simulink model "MultiVisualLocalizationAgent"  (R2024b)
settings: Solver=FixedStepAuto  StartTime=0.0  StopTime=inf  FixedStep=0.005  RelTol=1e-3  EnableMultiTasking=on
undefined symbols (not defined in the file or in its folder): gray, Sim3dSensor
libraries: eeGeneralControl x7, robotcorelib x7, dspstat3 x3, sim3dcameralib x2, uavsim3dlib x2, sim3dlib x1, uavutilslib x1
settings Model: Creator=The MathWorks, Inc.  LastModifiedBy=vince
settings SolverCC: AlgebraicLoopSolver=TrustRegion  PositivePriorityOrder=on  AutoInsertRateTranBlk=on  MaxZcPerStep=1
settings OptimizationCC: DefaultParameterBehavior=Inlined  EnhancedBackFolding=on  PassReuseOutputArgsAs=Individual arguments  ZeroExternalMemoryAtStartup=off  ZeroInternalMemoryAtStartup=off  MaxStackSize=200000  OptimizeBlockOrder=speed  DifferentSizesBufferReuse=on  OptimizationCustomize=off  EfficientTunableParamExpr=on
settings DebuggingCC: ParameterTunabilityLossMsg=error  UnconnectedInputMsg=warning  UnconnectedOutputMsg=warning  UnconnectedLineMsg=warning  SymbolicDimsDataTypeCodeGenerationDiagnostic=none
settings HardwareCC: ProdBitPerPointer=32  ProdBitPerSizeT=32  ProdBitPerPtrDiffT=32  ProdLargestAtomicInteger=Long  ProdLargestAtomicFloat=Double  ProdWordSize=32  ProdLongLongMode=on  ProdHWDeviceType=ARM Compatible->ARM Cortex-A (32-bit)
settings ModelReferenceCC: EnableRefExpFcnMdlSchedulingChecks=on
settings RTWCC: Description=Embedded Coder  SystemTargetFile=ert.tlc  HardwareBoard=Raspberry Pi  TLCOptions="-aInlineSetEventsForThisBaseRateFcn=TLC_FALSE -aSuppressMultiTaskScheduler=TLC_FALSE  -aRateBasedStepFcn=0"  TemplateMakefile=ert_default_tmf  Toolchain=GNU GCC Embedded Linux  BuildConfiguration=Faster Runs  GPUComputeCapability=3.5  DLArmComputeVersion=19.05
settings CodeAppCC: ForceParamTrailComments=on  IgnoreCustomStorageClasses=off  OperatorAnnotations=on  SimulinkDataObjDesc=on  SFDataObjDesc=on  InsertBlockDesc=on
settings ERTTargetCC: CodeReplacementLibrary=ARM Cortex-A CMSIS  SupportVariableSizeSignals=on  ExtModeTransport=2  ExtModeStaticAlloc=on  ExtModeMexFile=ext_xcp  ExtModeIntrfLevel=Level2 - Open

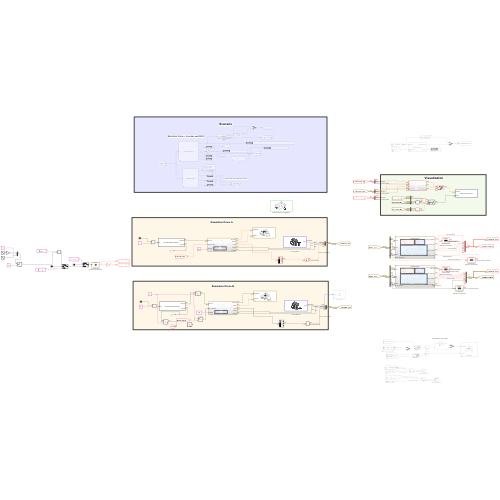
[thumbnail: Simulink's stored preview of the top-level diagram]
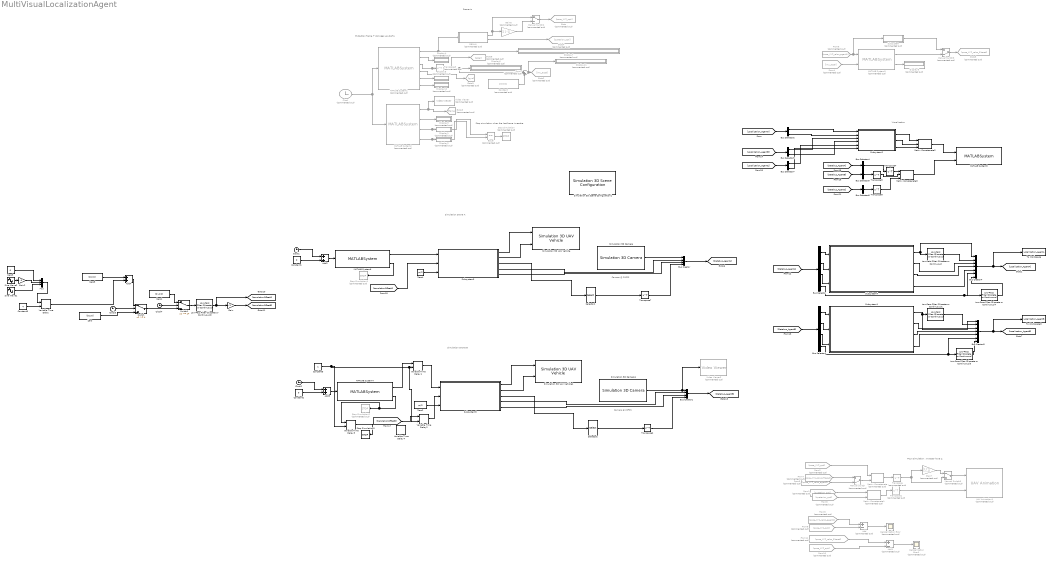
== system MultiVisualLocalizationAgent ==
  note: Stop simulation when the last frame is reache
  note: Pour Simulation : Inverser l'axe Z
  note: Extraction frame + données uavDATA
  note: Scenario
  note: Visualization
  note: Camera @ 20FPS
  note: Simulation Drone A
  note: Camera @ 20FPS
  note: Simulation Drone B
  Add : Sum  Commented=on  Inputs=+-
  Add1 : Sum  Commented=on  Inputs=+-
  Add2 : Sum
  Add3 : Sum
  Add4 : Sum
  Bus Creator : BusCreator  Inputs=4
  Bus Creator1 : BusCreator  Inputs=4
  Bus Creator3 : BusCreator  Inputs=7
  Bus Creator4 : BusCreator  Inputs=7
  Bus Selector : BusSelector  OutputSignals=accel,gyro,frame,Pose_XYZ_GroundTruth
  Bus Selector1 : BusSelector  OutputSignals=accel,gyro,frame,Pose_XYZ_GroundTruth
  Bus Selector2 : BusSelector  OutputSignals=Rotation_Mat_Reloc,Pose_XYZ_Kalman_Filtered
  Bus Selector3 : BusSelector  OutputSignals=Rotation_Mat_Reloc,Pose_XYZ_Kalman_Filtered
  Bus Selector4 : BusSelector  OutputSignals=Pose_XYZ_GroundTruth
  Bus Selector5 : BusSelector  OutputSignals=Pose_XYZ_GroundTruth
  Bus Selector7 : BusSelector  OutputSignals=Rotation_Mat_Reloc,Pose_XYZ_Kalman_Filtered
  Bus Selector8 : BusSelector  OutputSignals=Pose_XYZ_GroundTruth
  Clock : Clock  Commented=on
  Clock{1..4} (4 alike) : Clock
  Constant : Constant  Commented=on  Value=[0 0 0]
  Constant1 : Constant  Value=0
  Constant2 : Constant  Value=0
  Constant3 : Constant  Value=4
  Constant5 : Constant
  DEMUX : Subsystem  Commented=on
  Display{1..8,10..11} (10 alike) : Display  Commented=on
  Equal : RelationalOperator  Commented=on  Operator===  OutDataTypeStr=boolean  RndMeth=Simplest  InputSameDT=off
  From1 : From  Commented=on  GotoTag=quaterion_opti
  From10 : From  Commented=on  GotoTag=pose_XYZ_opti
  From11 : From  Commented=on  GotoTag=pose_XYZ_reloc_filtered
  From2 : From  Commented=on  GotoTag=pose_XYZ_opti
  From3 : From  Commented=on  GotoTag=pose_XYZ_reloc_agent1
  From4 : From  Commented=on  GotoTag=imu_accel
  From5 : From  Commented=on  GotoTag=quaterion_opti
  From6 : From  Commented=on  GotoTag=pose_XYZ_reloc_agent1
  From7 : From  Commented=on  GotoTag=pose_XYZ_reloc_filtered
  From8 : From  Commented=on  GotoTag=pose_XYZ_opti
  From9 : From  Commented=on  GotoTag=pose_XYZ_reloc_agent1
  Gain : Gain  Gain=-1
  Gain2 : Gain  Gain=-1
  Gain6 : Gain  Commented=on  Gain=[1 1 -1]
  Gain7 : Gain  Commented=on  Gain=[1 1 -1; 1 1 -1]
  Goto : Goto  Commented=on  GotoTag=pose_XYZ_opti
  Goto2 : Goto  Commented=on  GotoTag=imu_accel
  Goto3 : Goto  Commented=on  GotoTag=frame
  Goto4 : Goto  Commented=on  GotoTag=quaterion_opti
  Goto5 : Goto  Commented=on  GotoTag=pose_XYZ_reloc_filtered
  Goto8 : Goto  Commented=on  GotoTag=accel
  Goto9 : Goto  Commented=on  GotoTag=gyro
  Low-Pass Filter (Discrete or Continuous){,1,3..4} (4 alike) : eeGeneralControl/Low-Pass Filter (Discrete or Continuous)  K=1  T=0.5  B=inf  A=-inf  init_option=Inherited from block input  x0=0  Ts=-1
  Low-Pass Filter (Discrete or Continuous)2 : eeGeneralControl/Low-Pass Filter (Discrete or Continuous)  K=1  T=1  B=inf  A=-inf  init_option=Inherited from block input  x0=0  Ts=-1
  MATLAB System1 : MATLABSystem  Commented=on  System=GTruthPlayerSystem  groundTruthFile=C:\Users\vince\Documents\SEN5\CollaborativeSLAM\Scenarios\7\uavData.mat  SimulateUsing=Interpreted execution
      mask Type: GTruthPlayerSystem
      mask Display: disp('GTruthPlayerSystem');
  MATLAB System2 : MATLABSystem  Commented=on  System=ImagePlayerSystem  imageFolder=C:\Users\vince\Documents\SEN5\CollaborativeSLAM\Scenarios\7\images  cameraSize=[720,1280, 1]  groundTruthFile=C:\Users\vince\Documents\SEN5\CollaborativeSLAM\Scenarios\7\uavData.mat  SimulateUsing=Interpreted execution
      mask Type: ImagePlayerSystem
      mask Display: disp('ImagePlayerSystem');
  MATLAB System3 : MATLABSystem  Commented=on  System=PositionAccelFilter  maxPositionJump=0.2  maxAcceleration=10.0  windowSize=5  alpha=0.1  SimulateUsing=Code generation
      mask Type: PositionAccelFilter
      mask Display:
      | disp('PositionAccelFilter');
      | port_label('input',1,'position');
      | port_label('input',2,'acceleration');
      | port_label('output',1,'filteredPosition');
      | port_label('output',2,'isJump');
  MATLAB System4 : MATLABSystem  System=SmoothBasicWaypointManager  ScenariosDirectory=C:\Users\vince\Documents\SEN5\CollaborativeSLAM\Scenarios  ScenarioName=6  StepTime=0.01  SimulateUsing=Interpreted execution
      mask Type: SmoothBasicWaypointManager
      mask Display:
      | disp('SmoothBasicWaypointManager');
      | port_label('input',1,'time');
      | port_label('output',1,'waypoint');
      | port_label('output',2,'finished');
  MATLAB System5 : MATLABSystem  System=HelperVisualizationSystem  XLim=[-10 60]  YLim=[-10 10]  ZLim=[-10 10]  SampleTime=-1  ScenariosDirectory=C:\Users\vince\Documents\SEN5\CollaborativeSLAM\Scenarios  ScenarioName=8  NumberOfPoses=3  SimulateUsing=Interpreted execution
      mask Type: HelperVisualizationSystem
      mask Display:
      | disp('HelperVisualizationSystem');
      | port_label('input',1,'TformID');
      | port_label('input',2,'Gtruth');
  MATLAB System6 : MATLABSystem  System=SmoothBasicWaypointManager  ScenariosDirectory=C:\Users\vince\Documents\SEN5\CollaborativeSLAM\Scenarios  ScenarioName=6  StepTime=0.01  SimulateUsing=Interpreted execution
      mask Type: SmoothBasicWaypointManager
      mask Display:
      | disp('SmoothBasicWaypointManager');
      | port_label('input',1,'time');
      | port_label('output',1,'waypoint');
      | port_label('output',2,'finished');
  Manual Switch : ManualSwitch  Commented=on  CurrentSetting=0
  Manual Switch2 : ManualSwitch  Commented=on
  Manual Switch3 : ManualSwitch  Commented=on  CurrentSetting=0
  Manual Switch5 : ManualSwitch  Commented=on
  Matrix Concatenate : Concatenate  Commented=on  Mode=Multidimensional array  ConcatenateDimension=2
  Matrix Concatenate1 : Concatenate  Commented=on  Mode=Multidimensional array  ConcatenateDimension=2
  Matrix Concatenate2 : Concatenate  NumInputs=3  Mode=Multidimensional array  ConcatenateDimension=2
  Matrix Concatenate3 : Concatenate  NumInputs=3  Mode=Multidimensional array  ConcatenateDimension=2
  Mux : Mux  Inputs=3
  Relocalization Error : Scope  Commented=on
  Relocalization Error1 : Scope  Commented=on
  Selector1 : Selector  InputPortWidth=7  IndexOptions=Index vector (dialog)  Indices=[1 2 3]  OutputSizes=1
  Selector2 : Selector  InputPortWidth=7  IndexOptions=Index vector (dialog)  Indices=[1 2 3]  OutputSizes=1
  Simulation 3D Camera : sim3dcameralib/Simulation 3D Camera  Priority=1  sensorTag=Sim3dSensor�  sensorId=1  sensorName=Sim3dSensor�  vehTagList={'Scene Origin';'SimulinkVehicle1'}  vehTag=SimulinkVehicle1  mountLoc=Origin  offsetFlag=on  tmountOffset=[0.1, 0, 0.1]  extTmount=off  rmountOffset=[0, 0, 0]  extRmount=off  FocalLength=[1109, 1109]  OpticalCenter=[640, 360]  ImageSize=[720, 1280]  RadialDistortion=[0, 0]  TangentialDistortion=[0, 0]  SensorSkew=0  DepthOutportEnabled=off  SemanticOutportEnabled=off  TransformOutportEnabled=off  SampleTime=1/20  mountPoint=[0.1 0 0.1]  mountOrientation=[0 0 0]  aMode=3  ID=1
      settings: LibrarySourceBlock=drivingsim3d/Simulation 3D Camera
  Simulation 3D Camera1 : sim3dcameralib/Simulation 3D Camera  Priority=1  sensorTag=Sim3dSensor�  sensorId=2  sensorName=Sim3dSensor�  vehTagList={'Scene Origin';'SimulinkVehicle1';'SimulinkVehicle2'}  vehTag=SimulinkVehicle2  mountLoc=Origin  offsetFlag=on  tmountOffset=[0.1, 0, 0.1]  extTmount=off  rmountOffset=[0, 0, 0]  extRmount=off  FocalLength=[1109, 1109]  OpticalCenter=[640, 360]  ImageSize=[720, 1280]  RadialDistortion=[0, 0]  TangentialDistortion=[0, 0]  SensorSkew=0  DepthOutportEnabled=off  SemanticOutportEnabled=off  TransformOutportEnabled=off  SampleTime=1/20  mountPoint=[0.1 0 0.1]  mountOrientation=[0 0 0]  aMode=3  ID=2
      settings: LibrarySourceBlock=drivingsim3d/Simulation 3D Camera
  Simulation 3D Scene Configuration1 : sim3dlib/Simulation 3D Scene Configuration  Priority=0  ProjectFormat=Default Scenes  SceneDesc=US city block  ProjectName=C:\Program Files\MATLAB\R2024b\toolbox\shared\sim3d_projects\automotive_project_windows\UE\WindowsNoEditor\VehicleSimulation.exe  ScenePath=/Game/Maps/USCityBlock  EnableOpenDRIVE=off  vehTagList={'Custom';'Scene Origin';'SimulinkVehicle1';'SimulinkVehicle2';'SimulinkVehicle3'}  vehTag=SimulinkVehicle1  FreeCameraInitialTranslation=[0, 0, 0]  FreeCameraDefaultInitialTranslation=[-6, 0, 2]  FreeCameraInitialRotation=[0, 0, 0]  FreeCameraDefaultInitialRotation=[0, -15, 0]  OpVisEn=off  Ts=1/100  EnableWindow=off  EnableRemoteAccess=off  EnableWeather=off  SunAzimuth=90  SunAltitude=40.0  EnableGeospatialSun=off  Latitude=0  Longitude=0  Date=2023-01-01  Time=10:30:00  GeoTimeZone=-5.0  SunDaylightSaving=off  wind=1  clouds=10  EnableVolumetricClouds=off  CloudCoverage=0  CloudAltitude=6  fog=0  rain=0  RaindropsEffect=off  SnowDensity=0  EnableGeospatial=off  UseTrueOrigin=off  OriginHeight=200  OriginLatitude=40.744652  OriginLongitude=-73.988864  MapStyle=Aerial  AdditionalAssetIDs=[]  UseAdvancedSunSky=off  SolarTime=11  TimeZone=-5  Day=21  Month=9  Year=2022  UseDaylightSavingTime=on  DSTStartDay=10  DSTStartMonth=3  DSTEndDay=3  DSTEndMonth=11  DSTSwitchHour=2  sensorTag=MainCamera1  sensorId=1  sensorName=MainCamera1  mountLoc=Origin  offsetFlag=off  tmountOffset=[0, 0, 0]  rmountOffset=[0, 0, 0]  HorizontalResolution=1280  VerticalResolution=720  HorizontalFOV=60  mountPoint=[0 0 0]  mountOrientation=[0 0 0]  aMode=4  ID=1  GeoTrigger=Inactive
      settings: LibrarySourceBlock=uavsim3dlib/Simulation 3D Scene Configuration
  Simulation 3D UAV Vehicle : uavsim3dlib/Simulation 3D UAV Vehicle  Priority=-1  Mesh=Quadrotor  MeshPath=/MathWorksUAVContent/UAVs/HexaRotorUAV/HexaRotor.HexaRotor  Color=Black  ActorName=SimulinkVehicle1  UseGlobalFrame=off  InitialTranslation=[0 0 0]  InitialRotation=[0 0 0]  InitialTranslationGlobal=[0 0 0]  InitialGeoOrigin=[0 0 0]  InitialRotationGlobal=[0 0 0]  SampleTime=1/100  ActorType=SimulinkVehicle  ID=1  aMode=4  ActorTag=SimulinkVehicle1
  Simulation 3D UAV Vehicle1 : uavsim3dlib/Simulation 3D UAV Vehicle  Priority=-1  Mesh=Quadrotor  MeshPath=/MathWorksUAVContent/UAVs/HexaRotorUAV/HexaRotor.HexaRotor  Color=Black  ActorName=SimulinkVehicle2  UseGlobalFrame=off  InitialTranslation=[0 -2 0]  InitialRotation=[0 0 0]  InitialTranslationGlobal=[0 0 0]  InitialGeoOrigin=[0 0 0]  InitialRotationGlobal=[0 0 0]  SampleTime=1/100  ActorType=SimulinkVehicle  ID=2  aMode=4  ActorTag=SimulinkVehicle2
  Sine Wave1 : Sin  Frequency=2*pi/20  SampleTime=0
  Sine Wave2 : Sin  Amplitude=4  Frequency=2*pi/40  SampleTime=0
  Stop Simulation : Stop  Commented=on
  Stop Simulation1 : Stop  Commented=on
  Stop Simulation2 : Stop  Commented=on
  Stop Simulation3 : Stop
  Subsystem : Subsystem  Commented=on
  Subsystem1 : Subsystem  ReferencedSubsystem=LocalizationSystem
  Subsystem2 : Subsystem
  Subsystem3 : Subsystem
  Subsystem4 : Subsystem  ReferencedSubsystem=LocalizationSystem
  Subsystem5 : Subsystem
  Sum1 : Sum  Commented=on  Inputs=|++
  Switch : Switch  Threshold=4  SaturateOnIntegerOverflow=off  InputSameDT=off
  Switch1 : Switch  Threshold=14  SaturateOnIntegerOverflow=off  InputSameDT=off
  To Workspace : ToWorkspace  VariableName=Localization_AgentA  SaveFormat=Timeseries  SampleTime=-1
  To Workspace3 : ToWorkspace  VariableName=Localization_AgentB  SaveFormat=Timeseries  SampleTime=-1
  Transpose : Math  Commented=on  Operator=transpose
  Transpose1 : Math  Commented=on  Operator=transpose
  Transpose{2,4..5,7..8} (5 alike) : Math  Operator=transpose
  Transpose3 : Math  Commented=on  Operator=transpose
  UAV Animation1 : uavutilslib/UAV Animation  Commented=on  NumUAV=2  DynamicUAVConfig=off  UAVType=Multirotor  UAVSize=0.1  UAVColor=[1 0 0]  UAVTrajectoryAlpha=1  InertialZDirection=Down  RotationFormat=Quaternion  DrawMarkers=off  SampleTime=-1
  Variable Time Delay{,1..4} (5 alike) : VariableTransportDelay  MaximumDelay=10
  Video Viewer : VideoViewer  Commented=on  colormapValue=gray(256)  FigPos=[184.333333333333 766.666666666667 706 510]
  Video Viewer2 : VideoViewer  Commented=on  FigPos=[1 1030 1920 930]
  Zero : Constant  Value=[0;2;0]  OutDataTypeStr=Inherit: Inherit via back propagation
  Zero1 : Constant  Value=[0;-2;0]  OutDataTypeStr=Inherit: Inherit via back propagation
  Zero2 : Constant  Value=-pi/2  OutDataTypeStr=Inherit: Inherit via back propagation
  Zero3 : Constant  Value=0  OutDataTypeStr=Inherit: Inherit via back propagation
  Zero4 : Constant  Value=-pi/2  OutDataTypeStr=Inherit: Inherit via back propagation
  Zero5 : Constant  Value=[0;2;0]  OutDataTypeStr=Inherit: Inherit via back propagation
  wires:
  MATLAB System2/1 -> Goto3/1, Video Viewer/1
  MATLAB System2/3 -> Equal/1, Display1/1
  Clock/1 -> MATLAB System2/1, MATLAB System1/1
  MATLAB System2/4 -> Equal/2, Display2/1
  MATLAB System2/2 -> Display3/1
  MATLAB System1/1 -> Display7/1, DEMUX/1(pose_refopti_gtruth)
  Matrix Concatenate/1 -> Transpose/1
  Matrix Concatenate1/1 -> Transpose1/1
  Transpose/1 -> Gain7/1, Manual Switch5/2
  Transpose1/1 -> UAV Animation1/2
  From3/1 -> Manual Switch/2
  DEMUX/1(XYZ_gtruth) -> Manual Switch2/1, Gain6/1
  MATLAB System1/2 -> Display4/1
  MATLAB System1/5 -> Display5/1
  MATLAB System1/6 -> Display10/1
  MATLAB System1/3 -> Goto8/1, Transpose3/1
  DEMUX/2(quaterion_gtruth) -> Goto4/1
  From1/1 -> Matrix Concatenate1/1
  From5/1 -> Matrix Concatenate1/2
  From4/1 -> MATLAB System3/2
  From6/1 -> Subsystem/1(In1), MATLAB System3/1
  From7/1 -> Manual Switch/1
  Manual Switch/1 -> Matrix Concatenate/2
  Transpose3/1 -> Sum1/1, Display6/1
  MATLAB System3/2 -> Display8/1
  Constant/1 -> Sum1/2
  Sum1/1 -> Display11/1, Goto2/1
  MATLAB System3/1 -> Manual Switch3/2
  Subsystem/1(Out1) -> Manual Switch3/1
  From2/1 -> Matrix Concatenate/1
  Gain6/1 -> Manual Switch2/2
  Manual Switch2/1 -> Goto/1
  From8/1 -> Add/2  "Real_Pose_XYZ"
  Add/1 -> Relocalization Error/1  "Relocalization Error"
  From9/1 -> Add/1  "Estimated_Pose_XYZ"
  Add1/1 -> Relocalization Error1/1  "Filtered Relocalization Error"
  From10/1 -> Add1/2  "Real_Pose_XYZ"
  From11/1 -> Add1/1  "Estimated_Pose_XYZ_Filtered"
  Manual Switch3/1 -> Goto5/1
  Equal/1 -> Stop Simulation/1
  Manual Switch5/1 -> UAV Animation1/1
  Gain7/1 -> Manual Switch5/1
  MATLAB System1/4 -> Goto9/1
  Bus Selector2/1 -> Subsystem2/1(In1)  "<Rotation_Mat_Reloc>"
  Bus Selector2/2 -> Subsystem2/2(In2)  "<Pose_XYZ_Kalman_Filtered>"
  Subsystem2/1(Out1) -> Matrix Concatenate2/1
  Subsystem2/2(Out2) -> Matrix Concatenate2/2
  Clock1/1 -> Add2/1
  Add2/1 -> MATLAB System6/1
  Subsystem3/4(accData) -> Bus Creator/2  "accel"
  MATLAB System6/1 -> Subsystem3/1(waypoint)
  [translationOffsetA] -> Subsystem3/2(translationOffset)
  Subsystem3/1(Translation) -> Simulation 3D UAV Vehicle/1
  Subsystem3/3(gTruth) -> Selector1/1
  Zero4/1 -> Subsystem3/3(initialYaw)
  Subsystem3/2(Rotation) -> Simulation 3D UAV Vehicle/2
  MATLAB System6/2 -> Stop Simulation1/1
  Constant1/1 -> Add2/2
  Subsystem3/5(gyroData) -> Bus Creator/3  "gyro"
  Simulation 3D Camera/1 -> Bus Creator/1  "frame"
  Bus Selector3/2 -> Subsystem2/4(In4)  "<Pose_XYZ_Kalman_Filtered>"
  Bus Selector3/1 -> Subsystem2/3(In3)  "<Rotation_Mat_Reloc>"
  Selector1/1 -> Transpose7/1
  Transpose7/1 -> Bus Creator/4  "Pose_XYZ_GroundTruth"
  Matrix Concatenate3/1 -> MATLAB System5/2
  Low-Pass Filter (Discrete or Continuous)/1 -> Bus Creator4/2  "Pose_XYZ_Kalman_Filtered"
  Subsystem4/1 -> Low-Pass Filter (Discrete or Continuous)/1, Bus Creator4/1  "Pose_XYZ_Kalman"
  Subsystem4/3 -> Bus Creator4/4  "Pose_XYZ_Reloc"
  Subsystem4/4 -> Bus Creator4/5  "Rotation_Mat_Reloc"
  Bus Selector/3 -> Subsystem4/3  "<frame>"
  Bus Selector/2 -> Subsystem4/2  "<gyro>"
  Bus Selector/1 -> Subsystem4/1  "<accel>"
  Bus Creator/1 -> [Databus_AgentA]
  [Databus_AgentA] -> Bus Selector/1
  Bus Selector1/2 -> Subsystem1/2  "<gyro>"
  Bus Selector1/3 -> Subsystem1/3  "<frame>"
  [Databus_AgentB] -> Bus Selector1/1
  Bus Selector1/1 -> Subsystem1/1  "<accel>"
  Bus Creator1/1 -> [Databus_AgentB]
  Subsystem5/4(accData) -> Bus Creator1/2  "accel"
  Subsystem5/3(gTruth) -> Selector2/1
  Clock2/1 -> Add3/1
  Subsystem5/5(gyroData) -> Bus Creator1/3  "gyro"
  Subsystem5/2(Rotation) -> Simulation 3D UAV Vehicle1/2
  MATLAB System4/2 -> Variable Time Delay3/1, Stop Simulation2/1
  Add3/1 -> MATLAB System4/1
  Zero2/1 -> Subsystem5/3(initialYaw)
  Constant2/1 -> Add3/2
  MATLAB System4/1 -> Variable Time Delay1/1
  Transpose2/1 -> Bus Creator1/4  "Pose_XYZ_GroundTruth"
  Subsystem5/1(Translation) -> Simulation 3D UAV Vehicle1/1
  Selector2/1 -> Transpose2/1
  Bus Creator4/1 -> To Workspace/1, [Localization_AgentA]  "AgentA"
  Bus Creator3/1 -> To Workspace3/1, [Localization_AgentB]  "AgentB"
  Subsystem1/4 -> Bus Creator3/5  "Rotation_Mat_Reloc"
  Subsystem1/3 -> Bus Creator3/4  "Pose_XYZ_Reloc"
  Low-Pass Filter (Discrete or Continuous)1/1 -> Bus Creator3/2  "Pose_XYZ_Kalman_Filtered"
  Subsystem1/1 -> Bus Creator3/1, Low-Pass Filter (Discrete or Continuous)1/1  "Pose_XYZ_Kalman"
  [Localization_AgentA] -> Bus Selector2/1
  [Localization_AgentB] -> Bus Selector3/1
  [Databus_AgentA] -> Bus Selector4/1
  Bus Selector4/1 -> Transpose4/1  "<Pose_XYZ_GroundTruth>"
  [Databus_AgentB] -> Bus Selector5/1
  Bus Selector5/1 -> Transpose5/1  "<Pose_XYZ_GroundTruth>"
  Transpose4/1 -> Matrix Concatenate3/1
  Transpose5/1 -> Matrix Concatenate3/2
  Matrix Concatenate2/1 -> MATLAB System5/1
  Subsystem1/2 -> Bus Creator3/3
  Subsystem4/2 -> Bus Creator4/3
  Clock3/1 -> Switch/2
  Zero/1 -> Switch/3
  Switch1/1 -> Low-Pass Filter (Discrete or Continuous)2/1
  Switch/1 -> Switch1/3
  Clock4/1 -> Switch1/2
  Zero1/1 -> Switch1/1
  Sine Wave1/1 -> Mux/3
  Zero3/1 -> Mux/1
  Zero5/1 -> Add4/1
  Add4/1 -> Switch/1
  Low-Pass Filter (Discrete or Continuous)2/1 -> [translationOffsetA], Gain/1
  Mux/1 -> Variable Time Delay/1
  Gain2/1 -> Mux/2
  Gain/1 -> [translationOffsetB]
  Sine Wave2/1 -> Gain2/1
  Constant3/1 -> Variable Time Delay/2
  Variable Time Delay/1 -> Add4/2
  Bus Selector1/4 -> Bus Creator3/6, Low-Pass Filter (Discrete or Continuous)3/1  "<Pose_XYZ_GroundTruth>"
  Low-Pass Filter (Discrete or Continuous)3/1 -> Bus Creator3/7  "Pose_XYZ_GroundTruth_Filtered"
  Bus Selector/4 -> Low-Pass Filter (Discrete or Continuous)4/1, Bus Creator4/6  "<Pose_XYZ_GroundTruth>"
  Low-Pass Filter (Discrete or Continuous)4/1 -> Bus Creator4/7  "Pose_XYZ_GroundTruth_Filtered"
  [translationOffsetB] -> Variable Time Delay2/1
  Variable Time Delay2/1 -> Subsystem5/2(translationOffset)
  Variable Time Delay1/1 -> Subsystem5/1(waypoint)
  Constant5/1 -> Variable Time Delay2/2, Variable Time Delay1/2, Variable Time Delay3/2
  Simulation 3D Camera1/1 -> Video Viewer2/1, Bus Creator1/1  "frame"
  Variable Time Delay3/1 -> Stop Simulation3/1
  [Localization_AgentC] -> Bus Selector7/1
  Bus Selector7/1 -> Subsystem2/5(In5)  "<Rotation_Mat_Reloc>"
  Bus Selector7/2 -> Subsystem2/6(In6)  "<Pose_XYZ_Kalman_Filtered>"
  Subsystem2/3(Out3) -> Matrix Concatenate2/3
  [Databus_AgentC] -> Bus Selector8/1
  Transpose8/1 -> Matrix Concatenate3/3
  Bus Selector8/1 -> Transpose8/1  "<Pose_XYZ_GroundTruth>"

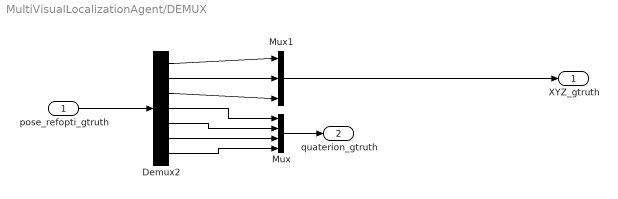
== system MultiVisualLocalizationAgent/DEMUX ==
  pose_refopti_gtruth : Inport
  Demux2 : Demux  Outputs=7
  Mux : Mux
  Mux1 : Mux  Inputs=3
  XYZ_gtruth : Outport
  quaterion_gtruth : Outport  Port=2
  wires:
  Mux/1 -> quaterion_gtruth/1
  Demux2/2 -> Mux1/2
  Demux2/5 -> Mux/2
  Mux1/1 -> XYZ_gtruth/1
  Demux2/3 -> Mux1/3
  Demux2/4 -> Mux/1
  pose_refopti_gtruth/1 -> Demux2/1
  Demux2/7 -> Mux/4
  Demux2/6 -> Mux/3
  Demux2/1 -> Mux1/1

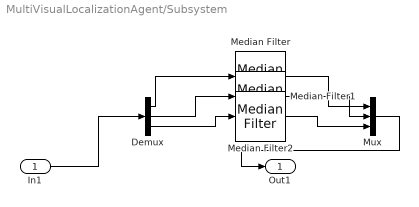
== system MultiVisualLocalizationAgent/Subsystem ==
  In1 : Inport
  Demux : Demux  Outputs=3
  Median Filter : dspstat3/Median Filter  WindowLength=2  SimulateUsing=Interpreted execution
  Median Filter1 : dspstat3/Median Filter  WindowLength=2  SimulateUsing=Interpreted execution
  Median Filter2 : dspstat3/Median Filter  WindowLength=2  SimulateUsing=Interpreted execution
  Mux : Mux  Inputs=3
  Out1 : Outport  PortDimensions=[3 1]
  wires:
  Median Filter2/1 -> Mux/3
  In1/1 -> Demux/1
  Demux/3 -> Median Filter2/1
  Mux/1 -> Out1/1
  Demux/2 -> Median Filter1/1
  Demux/1 -> Median Filter/1
  Median Filter1/1 -> Mux/2
  Median Filter/1 -> Mux/1

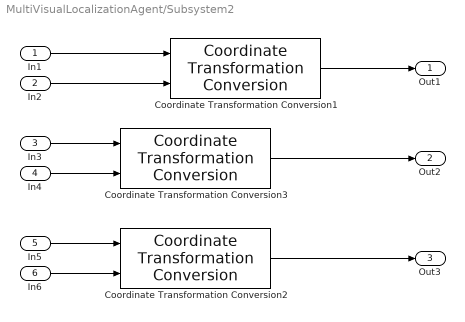
== system MultiVisualLocalizationAgent/Subsystem2 ==
  In1 : Inport
  In2 : Inport  Port=2
  In3 : Inport  Port=3
  In4 : Inport  Port=4
  In5 : Inport  Port=5
  In6 : Inport  Port=6
  Coordinate Transformation Conversion1 : robotcorelib/Coordinate Transformation Conversion  InputRepresentation=Rotation Matrix  InputEulerSequence=ZYX  ShowTrVecInputPort=on  OutputRepresentation=Homogeneous Transformation  OutputEulerSequence=ZYX  ShowTrVecOutputPort=on  SimulateUsing=Code generation
      settings: LibrarySourceBlock=navlib/Utilities/Coordinate Transformation Conversion
  Coordinate Transformation Conversion2 : robotcorelib/Coordinate Transformation Conversion  InputRepresentation=Rotation Matrix  InputEulerSequence=ZYX  ShowTrVecInputPort=on  OutputRepresentation=Homogeneous Transformation  OutputEulerSequence=ZYX  ShowTrVecOutputPort=on  SimulateUsing=Code generation
      settings: LibrarySourceBlock=navlib/Utilities/Coordinate Transformation Conversion
  Coordinate Transformation Conversion3 : robotcorelib/Coordinate Transformation Conversion  InputRepresentation=Rotation Matrix  InputEulerSequence=ZYX  ShowTrVecInputPort=on  OutputRepresentation=Homogeneous Transformation  OutputEulerSequence=ZYX  ShowTrVecOutputPort=on  SimulateUsing=Code generation
      settings: LibrarySourceBlock=navlib/Utilities/Coordinate Transformation Conversion
  Out1 : Outport
  Out2 : Outport  Port=2
  Out3 : Outport  Port=3
  wires:
  Coordinate Transformation Conversion3/1 -> Out2/1
  In3/1 -> Coordinate Transformation Conversion3/1
  Coordinate Transformation Conversion1/1 -> Out1/1
  In1/1 -> Coordinate Transformation Conversion1/1
  In4/1 -> Coordinate Transformation Conversion3/2
  In2/1 -> Coordinate Transformation Conversion1/2
  In6/1 -> Coordinate Transformation Conversion2/2
  In5/1 -> Coordinate Transformation Conversion2/1
  Coordinate Transformation Conversion2/1 -> Out3/1

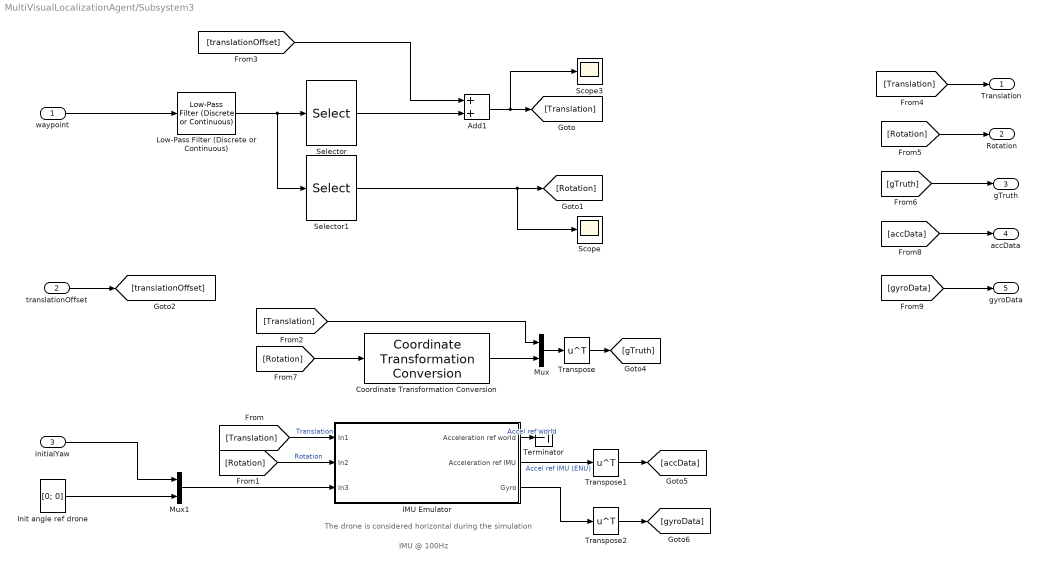
== system MultiVisualLocalizationAgent/Subsystem3 ==
  note: IMU @ 100Hz
  note: The drone is considered horizontal during the simulation
  waypoint : Inport
  translationOffset : Inport  Port=2
  initialYaw : Inport  Port=3
  Add1 : Sum
  Coordinate Transformation Conversion : robotcorelib/Coordinate Transformation Conversion  InputRepresentation=Euler Angles  InputEulerSequence=ZYX  ShowTrVecInputPort=on  OutputRepresentation=Quaternion  OutputEulerSequence=ZYX  ShowTrVecOutputPort=on  SimulateUsing=Code generation
  IMU Emulator : Subsystem
  Init angle ref drone : Constant  Value=[0; 0]  VectorParams1D=off
  Low-Pass Filter (Discrete or Continuous) : eeGeneralControl/Low-Pass Filter (Discrete or Continuous)  K=1  T=0.5  B=inf  A=-inf  init_option=Inherited from block input  x0=0  Ts=-1
  Mux : Mux  Inputs=2
  Mux1 : Mux  Inputs=2
  Scope : Scope
  Scope3 : Scope
  Selector : Selector  InputPortWidth=6  IndexOptions=Index vector (dialog)  Indices=[1 2 3]  OutputSizes=1
  Selector1 : Selector  InputPortWidth=6  IndexOptions=Index vector (dialog)  Indices=[4 5 6]  OutputSizes=1
  Terminator : Terminator
  Transpose : Math  Operator=transpose
  Transpose1 : Math  Operator=transpose
  Transpose2 : Math  Operator=transpose
  Translation : Outport
  Rotation : Outport  Port=2
  gTruth : Outport  Port=3
  accData : Outport  Port=4
  gyroData : Outport  Port=5
  wires:
  waypoint/1 -> Low-Pass Filter (Discrete or Continuous)/1
  Add1/1 -> Scope3/1, [Translation]
  Transpose2/1 -> [gyroData]
  Selector/1 -> Add1/2
  Init angle ref drone/1 -> Mux1/2
  Selector1/1 -> [Rotation], Scope/1
  IMU Emulator/3(Gyro) -> Transpose2/1
  Coordinate Transformation Conversion/1 -> Mux/2
  IMU Emulator/1(Acceleration ref world) -> Terminator/1  "Accel ref world"
  [translationOffset] -> Add1/1
  Mux/1 -> Transpose/1
  [Rotation] -> Coordinate Transformation Conversion/1
  Transpose1/1 -> [accData]
  Transpose/1 -> [gTruth]
  [Translation] -> Mux/1
  Low-Pass Filter (Discrete or Continuous)/1 -> Selector1/1, Selector/1
  [Rotation] -> IMU Emulator/2(In2)  "Rotation"
  [Translation] -> IMU Emulator/1(In1)  "Translation"
  IMU Emulator/2(Acceleration ref IMU) -> Transpose1/1  "Accel ref IMU (ENU)"
  [Translation] -> Translation/1
  [Rotation] -> Rotation/1
  [gTruth] -> gTruth/1
  [accData] -> accData/1
  [gyroData] -> gyroData/1
  initialYaw/1 -> Mux1/1
  Mux1/1 -> IMU Emulator/3(In3)
  translationOffset/1 -> [translationOffset]

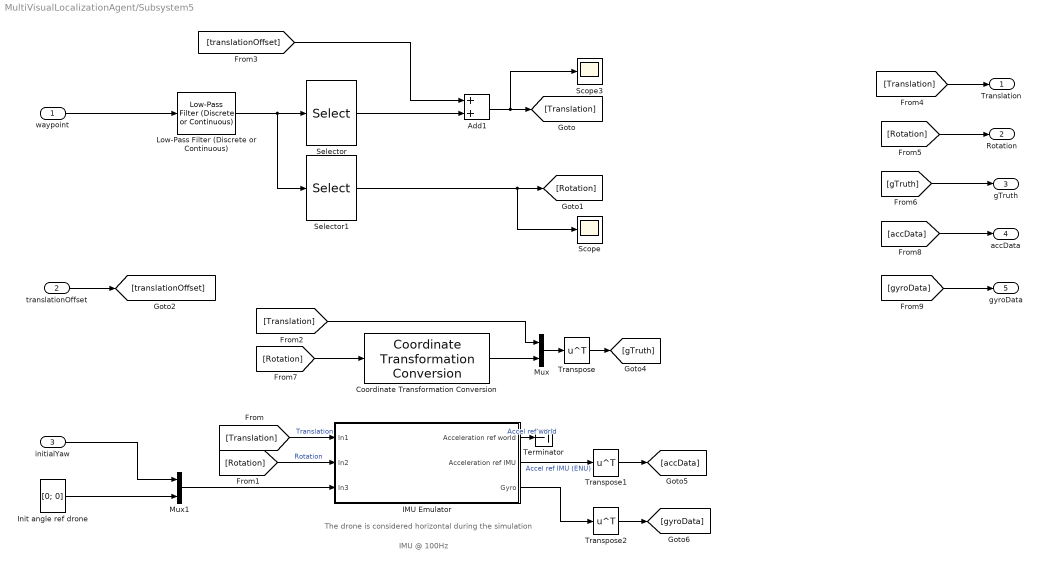
== system MultiVisualLocalizationAgent/Subsystem5 ==
  note: IMU @ 100Hz
  note: The drone is considered horizontal during the simulation
  waypoint : Inport
  translationOffset : Inport  Port=2
  initialYaw : Inport  Port=3
  Add1 : Sum
  Coordinate Transformation Conversion : robotcorelib/Coordinate Transformation Conversion  InputRepresentation=Euler Angles  InputEulerSequence=ZYX  ShowTrVecInputPort=on  OutputRepresentation=Quaternion  OutputEulerSequence=ZYX  ShowTrVecOutputPort=on  SimulateUsing=Code generation
  IMU Emulator : Subsystem
  Init angle ref drone : Constant  Value=[0; 0]  VectorParams1D=off
  Low-Pass Filter (Discrete or Continuous) : eeGeneralControl/Low-Pass Filter (Discrete or Continuous)  K=1  T=0.5  B=inf  A=-inf  init_option=Inherited from block input  x0=0  Ts=-1
  Mux : Mux  Inputs=2
  Mux1 : Mux  Inputs=2
  Scope : Scope
  Scope3 : Scope
  Selector : Selector  InputPortWidth=6  IndexOptions=Index vector (dialog)  Indices=[1 2 3]  OutputSizes=1
  Selector1 : Selector  InputPortWidth=6  IndexOptions=Index vector (dialog)  Indices=[4 5 6]  OutputSizes=1
  Terminator : Terminator
  Transpose : Math  Operator=transpose
  Transpose1 : Math  Operator=transpose
  Transpose2 : Math  Operator=transpose
  Translation : Outport
  Rotation : Outport  Port=2
  gTruth : Outport  Port=3
  accData : Outport  Port=4
  gyroData : Outport  Port=5
  wires:
  waypoint/1 -> Low-Pass Filter (Discrete or Continuous)/1
  Add1/1 -> Scope3/1, [Translation]
  Transpose2/1 -> [gyroData]
  Selector/1 -> Add1/2
  Init angle ref drone/1 -> Mux1/2
  Selector1/1 -> [Rotation], Scope/1
  IMU Emulator/3(Gyro) -> Transpose2/1
  Coordinate Transformation Conversion/1 -> Mux/2
  IMU Emulator/1(Acceleration ref world) -> Terminator/1  "Accel ref world"
  [translationOffset] -> Add1/1
  Mux/1 -> Transpose/1
  [Rotation] -> Coordinate Transformation Conversion/1
  Transpose1/1 -> [accData]
  Transpose/1 -> [gTruth]
  [Translation] -> Mux/1
  Low-Pass Filter (Discrete or Continuous)/1 -> Selector1/1, Selector/1
  [Rotation] -> IMU Emulator/2(In2)  "Rotation"
  [Translation] -> IMU Emulator/1(In1)  "Translation"
  IMU Emulator/2(Acceleration ref IMU) -> Transpose1/1  "Accel ref IMU (ENU)"
  [Translation] -> Translation/1
  [Rotation] -> Rotation/1
  [gTruth] -> gTruth/1
  [accData] -> accData/1
  [gyroData] -> gyroData/1
  initialYaw/1 -> Mux1/1
  Mux1/1 -> IMU Emulator/3(In3)
  translationOffset/1 -> [translationOffset]

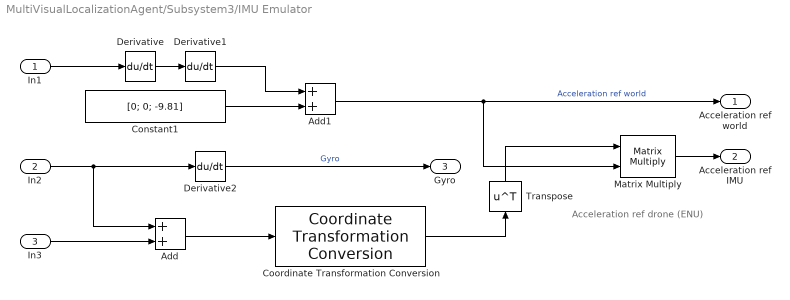
== system MultiVisualLocalizationAgent/Subsystem3/IMU Emulator ==
  note: Acceleration ref drone (ENU)
  In1 : Inport
  In2 : Inport  Port=2
  In3 : Inport  Port=3
  Add : Sum
  Add1 : Sum
  Constant1 : Constant  Value=[0; 0; -9.81]
  Coordinate Transformation Conversion : robotcorelib/Coordinate Transformation Conversion  InputRepresentation=Euler Angles  InputEulerSequence=ZYX  ShowTrVecInputPort=on  OutputRepresentation=Rotation Matrix  OutputEulerSequence=ZYX  ShowTrVecOutputPort=on  SimulateUsing=Code generation
  Derivative : Derivative
  Derivative1 : Derivative
  Derivative2 : Derivative
  Matrix Multiply : Product  Multiplication=Matrix(*)
  Transpose : Math  Operator=transpose
  Acceleration ref world : Outport
  Acceleration ref IMU : Outport  Port=2
  Gyro : Outport  Port=3
  wires:
  Derivative/1 -> Derivative1/1
  Derivative2/1 -> Gyro/1  "Gyro"
  Constant1/1 -> Add1/2
  Add1/1 -> Matrix Multiply/2, Acceleration ref world/1  "Acceleration ref world"
  Derivative1/1 -> Add1/1
  In1/1 -> Derivative/1
  In2/1 -> Add/1, Derivative2/1
  In3/1 -> Add/2
  Add/1 -> Coordinate Transformation Conversion/1
  Matrix Multiply/1 -> Acceleration ref IMU/1
  Coordinate Transformation Conversion/1 -> Transpose/1
  Transpose/1 -> Matrix Multiply/1

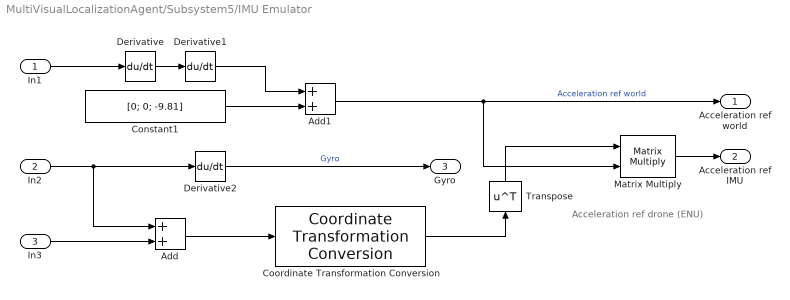
== system MultiVisualLocalizationAgent/Subsystem5/IMU Emulator ==
  note: Acceleration ref drone (ENU)
  In1 : Inport
  In2 : Inport  Port=2
  In3 : Inport  Port=3
  Add : Sum
  Add1 : Sum
  Constant1 : Constant  Value=[0; 0; -9.81]
  Coordinate Transformation Conversion : robotcorelib/Coordinate Transformation Conversion  InputRepresentation=Euler Angles  InputEulerSequence=ZYX  ShowTrVecInputPort=on  OutputRepresentation=Rotation Matrix  OutputEulerSequence=ZYX  ShowTrVecOutputPort=on  SimulateUsing=Code generation
  Derivative : Derivative
  Derivative1 : Derivative
  Derivative2 : Derivative
  Matrix Multiply : Product  Multiplication=Matrix(*)
  Transpose : Math  Operator=transpose
  Acceleration ref world : Outport
  Acceleration ref IMU : Outport  Port=2
  Gyro : Outport  Port=3
  wires:
  Derivative/1 -> Derivative1/1
  Derivative2/1 -> Gyro/1  "Gyro"
  Constant1/1 -> Add1/2
  Add1/1 -> Matrix Multiply/2, Acceleration ref world/1  "Acceleration ref world"
  Derivative1/1 -> Add1/1
  In1/1 -> Derivative/1
  In2/1 -> Add/1, Derivative2/1
  In3/1 -> Add/2
  Add/1 -> Coordinate Transformation Conversion/1
  Matrix Multiply/1 -> Acceleration ref IMU/1
  Coordinate Transformation Conversion/1 -> Transpose/1
  Transpose/1 -> Matrix Multiply/1
